simulink model "Speed_Controller_Test_gr3"  (Simulink 7.0)
settings: Solver=ode4  SolverMode=SingleTasking  StartTime=0.0  StopTime=252  FixedStep=0.01  RelTol=1e-3
InitFcn:
  | tempomat_para
StopFcn:
  | clear;
values from neighbouring files (symbols this model uses):
  A = 1.9    [tempomat_para.m]
  a_Fzg_max = 2    [tempomat_para.m]
  a_Fzg_min = -2    [tempomat_para.m]
  cw = 0.32    [tempomat_para.m]
  gang = [1 2 3 4]    [tempomat_para.m]
  gang_vec = [1 2 3 4]    [tempomat_para.m]
  i_anteil = 5    [tempomat_para.m]
  i_d = 3.42    [tempomat_para.m]
  i_g = [3.91 2.17 1.37 1.00]    [tempomat_para.m]
  lambda_gang = [1.3 1.25  1.17  1.05]    [tempomat_para.m]
  m_Fzg = 1400    [tempomat_para.m]
  M_mot_max = [130 149 163 170 168 166 162 158 150 139 123 80]    [tempomat_para.m]
  M_mot_min = [0 -40]    [tempomat_para.m]
  n_mot0 = 1000    [tempomat_para.m]
  n_mot_max = 1000:500:6500    [tempomat_para.m]
  n_mot_min = [1000 6500]    [tempomat_para.m]
  p_anteil = 100    [tempomat_para.m]
  r_dyn = 0.28    [tempomat_para.m]
  rho = 1.202    [tempomat_para.m]
  t_sch = 0.2    [tempomat_para.m]
  TI = [block '/TI']    [PSTI_callback.m]
  v_Fzg_ms0 = 0    [tempomat_para.m]
undefined symbols (not defined in the file or in its folder): Drossel_mat, getdatatypespecs
libraries: simulink x284, fzgbib x6
(part 1 of 19)
settings Model: Creator=Abel  LastModifiedBy=jza
settings DataIOCC: LimitDataPoints=off  SignalLoggingName=sigsOut
settings OptimizationCC: BooleanDataType=off
settings DebuggingCC: SaveWithParameterizedLinksMsg=none  SignalResolutionControl=TryResolveAllWithWarning  InheritedTsInSrcMsg=none  MultiTaskDSMMsg=warning  MultiTaskCondExecSysMsg=none  StrictBusMsg=None
settings RTWCC: IncludeERTFirstTime=on
settings GRTTargetCC: TargetFcnLib=ansi_tfl_tmw.mat

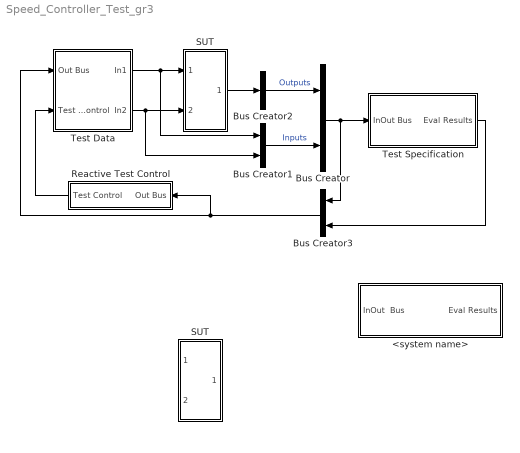
== system Speed_Controller_Test_gr3 ==
  <system name> : Subsystem  Description=Test evaluation system template. Create a new test evaluation system from this template.  mask{No=3, T=off}
      mask prompts: No "Number of Requirements"; T "Shut off the mask"
      mask StyleString: popup(1|2|3|4|5|6|7|8|9|10|11|12|13|14|15|16|17|18|19|20),checkbox
      mask CallbackString: system_name2(gcb);|shut_mask(gcb);
  Bus Creator : BusCreator  Inputs=2
  Bus Creator1 : BusCreator  Inputs=2
  Bus Creator2 : BusCreator  Inputs=1
  Bus Creator3 : BusCreator  Orientation=left  Inputs=2
  Reactive Test Control : Subsystem  Orientation=left
  SUT : Subsystem
  "SUT " : Subsystem
  Test Data : Subsystem
  Test Specification : Subsystem  Description=Test evaluation system template. Create a new test evaluation system from this template.
  wires:
  SUT/1(Out1) -> Bus Creator2/1
  Bus Creator/1 -> Test Specification/1(InOut Bus), Bus Creator3/1
  Bus Creator2/1 -> Bus Creator/1  "Outputs"
  Bus Creator1/1 -> Bus Creator/2  "Inputs"
  Bus Creator3/1 -> Test Data/1(Out Bus), Reactive Test Control/1(Out Bus)
  Test Specification/1(Eval Results) -> Bus Creator3/2
  Reactive Test Control/1(Test Control) -> Test Data/2(Test Control)
  Test Data/1(In1) -> SUT/1(In1), Bus Creator1/1
  Test Data/2(In2) -> SUT/2(In2), Bus Creator1/2

== system Speed_Controller_Test_gr3/<system name> ==
  InOut  Bus : Inport  OutDataType=sfix(16)  OutScaling=2^0
  <Requirement name> : Subsystem  Description=Requirement template. Create a new requirement from this template.  mask{No=1}
      mask prompts: No "Number of single Validation Functions"
      mask StyleString: popup(1|2|3|4|5|6|7|8|9|10|11|12|13|14|15|16|17|18|19|20)
      mask CallbackString: ReqName_callback(gcb);
  <Requirement name>2 : Subsystem  Description=Requirement template. Create a new requirement from this template.  mask{No=3}
      mask prompts: No "Number of single Validation Functions"
      mask StyleString: popup(1|2|3|4|5|6|7|8|9|10|11|12|13|14|15|16|17|18|19|20)
      mask CallbackString: ReqName_callback(gcb);
  <Requirement name>3 : Subsystem  Description=Requirement template. Create a new requirement from this template.  mask{No=2}
      mask prompts: No "Number of single Validation Functions"
      mask StyleString: popup(1|2|3|4|5|6|7|8|9|10|11|12|13|14|15|16|17|18|19|20)
      mask CallbackString: ReqName_callback(gcb);
  Arbitration : Subsystem
  Bus Creator : BusCreator  Inputs=3
  Bus Creator1 : BusCreator  Inputs=2
  Bus Creator4 : BusCreator  Inputs=6
  Bus Selector : BusSelector  OutputSignals=signal1.signal1.signal1,signal2.signal1.signal1,signal3.signal1.signal1,signal3.signal2.signal1,signal2.signal2.signal1,signal2.signal3.signal1
  Signal Conversion : SignalConversion  ConversionOutput=Bus copy
  Eval Results : Outport  OutDataType=sfix(16)  OutScaling=2^0
  wires:
  Bus Creator1/1 -> Eval Results/1
  Bus Creator4/1 -> Bus Creator1/2
  Signal Conversion/1 -> <Requirement name>/1(InOut Bus), <Requirement name>2/1(InOut Bus), <Requirement name>3/1(InOut Bus)
  InOut  Bus/1 -> Signal Conversion/1
  <Requirement name>/1(Test Info) -> Bus Creator/1
  Arbitration/1(OV) -> Bus Creator1/1
  <Requirement name>2/1(Test Info) -> Bus Creator/2
  <Requirement name>3/1(Test Info) -> Bus Creator/3
  Bus Creator/1 -> Bus Selector/1
  Bus Selector/1 -> Arbitration/1(v1), Bus Creator4/1  "<signal1>"
  Bus Selector/2 -> Arbitration/2(v2), Bus Creator4/2  "<signal1>"
  Bus Selector/3 -> Arbitration/3(v3), Bus Creator4/3  "<signal1>"
  Bus Selector/4 -> Arbitration/4(v4), Bus Creator4/4  "<signal1>"

== system Speed_Controller_Test_gr3/Reactive Test Control ==
  Out Bus : Inport  OutDataType=sfix(16)  OutScaling=2^0
  Bus Selector : BusSelector  OutputSignals=signal2.signal1.signal1.signal1.signal1.Local verdict
  Counter : Subsystem
  Memory : Memory
  OR : Logic  Operator=OR  Inputs=3  AllPortsSameDT=off  OutDataTypeMode=boolean
  Switch : Switch  Criteria=u2 > Threshold
  error : simulink/Logic and Bit Operations/Compare To Constant  SystemSampleTime=-1  relop===  const=-1  LogicOutDataTypeMode=uint8  ZeroCross=off
  fail : simulink/Logic and Bit Operations/Compare To Constant  SystemSampleTime=-1  relop===  const=0  LogicOutDataTypeMode=uint8  ZeroCross=off
  pass : simulink/Logic and Bit Operations/Compare To Constant  SystemSampleTime=-1  relop===  const=1  LogicOutDataTypeMode=uint8  ZeroCross=off
  test case 1 : Constant  OutDataType=sfix(16)  OutScaling=2^0
  test case 2 : Constant  Value=2  OutDataType=sfix(16)  OutScaling=2^0
  Test Control : Outport  OutDataType=sfix(16)  OutScaling=2^0
  wires:
  OR/1 -> Counter/1(In1), Counter/Trigger
  test case 1/1 -> Switch/3
  Out Bus/1 -> Bus Selector/1
  Switch/1 -> Test Control/1
  test case 2/1 -> Switch/1
  Counter/1(Out1) -> Switch/2
  Bus Selector/1 -> Memory/1  "<Local verdict>"
  pass/1 -> OR/1
  fail/1 -> OR/2
  error/1 -> OR/3
  Memory/1 -> pass/1, error/1, fail/1

== system Speed_Controller_Test_gr3/SUT ==
  In1 : Inport  OutDataType=sfix(16)  OutScaling=2^0
  In2 : Inport  Port=2  OutDataType=sfix(16)  OutScaling=2^0
  " Speed Controller " : Subsystem  AncestorBlock=fzgbib/GeschwindigkeitsRegelung
  Terminator1 : Terminator
  Terminator2 : Terminator
  Vehicle Model : Subsystem
      mask Type: Vehicle Model
      mask Display: image(imread('car.jpg','jpg'),[0.05,0.2,0.9,0.6])
  Out1 : Outport  OutDataType=sfix(16)  OutScaling=2^0
  wires:
  Vehicle Model/2(M_Br_b) -> Terminator1/1
  Vehicle Model/3(M_Mot_b) -> Terminator2/1
  " Speed Controller "/1(CarInputs) -> Vehicle Model/1(StellgroessenTempomat)
  Vehicle Model/1(FzgDaten) -> " Speed Controller "/1(CarOutputs)
  " Speed Controller "/2(v_act) -> Out1/1
  In2/1 -> " Speed Controller "/3(Selection)
  In1/1 -> " Speed Controller "/4(v_Des)

== system Speed_Controller_Test_gr3/SUT  ==
  In1 : Inport  OutDataType=sfix(16)  OutScaling=2^0
  In2 : Inport  Port=2  OutDataType=sfix(16)  OutScaling=2^0
  " Speed Controller " : Subsystem  AncestorBlock=fzgbib/GeschwindigkeitsRegelung
  Terminator1 : Terminator
  Terminator2 : Terminator
  Vehicle Model : Subsystem
      mask Type: Vehicle Model
      mask Display: image(imread('car.jpg','jpg'),[0.05,0.2,0.9,0.6])
  Out1 : Outport  OutDataType=sfix(16)  OutScaling=2^0
  wires:
  Vehicle Model/2(M_Br_b) -> Terminator1/1
  Vehicle Model/3(M_Mot_b) -> Terminator2/1
  " Speed Controller "/1(CarInputs) -> Vehicle Model/1(StellgroessenTempomat)
  Vehicle Model/1(FzgDaten) -> " Speed Controller "/1(CarOutputs)
  " Speed Controller "/2(v_act) -> Out1/1
  In2/1 -> " Speed Controller "/3(Selection)
  In1/1 -> " Speed Controller "/4(v_Des)

== system Speed_Controller_Test_gr3/Test Data ==
  Out Bus : Inport  OutDataType=sfix(16)  OutScaling=2^0
  Test Control : Inport  Port=2  OutDataType=sfix(16)  OutScaling=2^0
  Bus Creator : BusCreator  Inputs=6
  Bus Selector : BusSelector  OutputSignals=v_Des (signal 1),v_Des (signal 4)
  Bus Selector1 : BusSelector  OutputSignals=CCMode (signal 2),CCMode (signal 5)
  Bus Selector2 : BusSelector  OutputSignals=Selection (signal 3),Selection (signal 6)
  PrecAct CCMode : MultiPortSwitch  Inputs=3  zeroidx=on
  PrecAct Selection : MultiPortSwitch  Inputs=3  zeroidx=on
  PrecAct v_Des : MultiPortSwitch  Inputs=3  zeroidx=on
  R1 Speed Control step response : Subsystem
  R2 Speed Control velocity restoration time after simple  acceleration/deceleration : Subsystem
  zero signal : Constant  Value=0  OutDataType=sfix(16)  OutScaling=2^0
  In1 : Outport  OutDataType=sfix(16)  OutScaling=2^0
  In2 : Outport  Port=2  OutDataType=sfix(16)  OutScaling=2^0
  wires:
  Out Bus/1 -> R1 Speed Control step response/1(Out Bus)
  zero signal/1 -> PrecAct v_Des/2, PrecAct Selection/2, PrecAct CCMode/2
  PrecAct CCMode/1 -> In1/1
  PrecAct Selection/1 -> In2/1
  Bus Creator/1 -> Bus Selector/1, Bus Selector1/1, Bus Selector2/1
  Bus Selector/1 -> PrecAct v_Des/3  "<v_Des (signal 1)>"
  R1 Speed Control step response/1(v_Des) -> Bus Creator/1
  R1 Speed Control step response/2(CCMode) -> Bus Creator/2
  R1 Speed Control step response/3(Selection) -> Bus Creator/3
  R2 Speed Control velocity restoration time after simple  acceleration/deceleration/1(v_Des) -> Bus Creator/4
  R2 Speed Control velocity restoration time after simple  acceleration/deceleration/2(CCMode) -> Bus Creator/5
  R2 Speed Control velocity restoration time after simple  acceleration/deceleration/3(Selection) -> Bus Creator/6
  Bus Selector/2 -> PrecAct v_Des/4  "<v_Des (signal 4)>"
  Bus Selector1/1 -> PrecAct CCMode/3  "<CCMode (signal 2)>"
  Bus Selector1/2 -> PrecAct CCMode/4  "<CCMode (signal 5)>"
  Bus Selector2/1 -> PrecAct Selection/3  "<Selection (signal 3)>"
  Bus Selector2/2 -> PrecAct Selection/4  "<Selection (signal 6)>"
  Test Control/1 -> PrecAct v_Des/1, PrecAct CCMode/1, PrecAct Selection/1

== system Speed_Controller_Test_gr3/Test Specification ==
  InOut Bus : Inport  OutDataType=sfix(16)  OutScaling=2^0
  Arbitration : Subsystem
  Bus Creator1 : BusCreator  Inputs=2
  Bus Creator2 : BusCreator  Inputs=2
  Bus Selector1 : BusSelector  OutputSignals=signal1.signal1.signal1.Local verdict,signal1.signal1.signal2.Local verdict,signal2.signal1.signal1.Local verdict
  R1 Speed Control step response : Subsystem  Description=Requirement template. Create a new requirement from this template.
  R2 Speed Control velocity restoration time after simple  acceleration/deceleration : Subsystem  Description=Requirement template. Create a new requirement from this template.
  Signal Conversion : SignalConversion  ConversionOutput=Bus copy
  Eval Results : Outport  OutDataType=sfix(16)  OutScaling=2^0
  wires:
  Signal Conversion/1 -> R1 Speed Control step response/1(InOut Bus), R2 Speed Control velocity restoration time after simple  acceleration/deceleration/1(InOut Bus)
  R1 Speed Control step response/1(Test Info) -> Bus Creator2/1
  InOut Bus/1 -> Signal Conversion/1
  Bus Creator2/1 -> Bus Selector1/1, Bus Creator1/1
  R2 Speed Control velocity restoration time after simple  acceleration/deceleration/1(Test Info) -> Bus Creator2/2
  Bus Selector1/1 -> Arbitration/1(In1)  "<Local verdict>"
  Bus Selector1/2 -> Arbitration/2(In2)  "<Local verdict>"
  Bus Selector1/3 -> Arbitration/3(In3)  "<Local verdict>"
  Bus Creator1/1 -> Eval Results/1
  Arbitration/1(Out1) -> Bus Creator1/2  "Overall verdict"

== system Speed_Controller_Test_gr3/<system name>/<Requirement name> ==
  InOut Bus : Inport  OutDataType=sfix(16)  OutScaling=2^0
  <Assertions name> : Subsystem  Description=Assertions template. Create a new assertions block from this template.
  <Preconditions name> : Subsystem  Description=Preconditions template. Create new preconditions blocks using this template.
  Bus Creator : BusCreator  Inputs=1
  Test Info : Outport  OutDataType=sfix(16)  OutScaling=2^0
  wires:
  <Preconditions name>/1(Activate) -> <Assertions name>/1(Precond)
  Bus Creator/1 -> Test Info/1
  <Assertions name>/1(VF info) -> Bus Creator/1
  InOut Bus/1 -> <Preconditions name>/1(InOut Bus), <Assertions name>/2(InOut Bus)

== system Speed_Controller_Test_gr3/<system name>/<Requirement name>2 ==
  InOut Bus : Inport  OutDataType=sfix(16)  OutScaling=2^0
  <Assertions name> : Subsystem  Description=Assertions template. Create a new assertions block from this template.
  <Assertions name>2 : Subsystem  Description=Assertions template. Create a new assertions block from this template.
  <Assertions name>3 : Subsystem  Description=Assertions template. Create a new assertions block from this template.
  <Preconditions name> : Subsystem  Description=Preconditions template. Create new preconditions blocks using this template.
  <Preconditions name>2 : Subsystem  Description=Preconditions template. Create new preconditions blocks using this template.
  <Preconditions name>3 : Subsystem  Description=Preconditions template. Create new preconditions blocks using this template.
  Bus Creator : BusCreator  Inputs=3
  Test Info : Outport  OutDataType=sfix(16)  OutScaling=2^0
  wires:
  <Preconditions name>/1(Activate) -> <Assertions name>/1(Precond)
  Bus Creator/1 -> Test Info/1
  <Assertions name>/1(VF info) -> Bus Creator/1
  InOut Bus/1 -> <Preconditions name>/1(InOut Bus), <Assertions name>/2(InOut Bus), <Assertions name>2/2(InOut Bus), <Preconditions name>2/1(InOut Bus), <Assertions name>3/2(InOut Bus), <Preconditions name>3/1(InOut Bus)
  <Preconditions name>2/1(Activate) -> <Assertions name>2/1(Precond)
  <Assertions name>2/1(VF info) -> Bus Creator/2
  <Preconditions name>3/1(Activate) -> <Assertions name>3/1(Precond)
  <Assertions name>3/1(VF info) -> Bus Creator/3

== system Speed_Controller_Test_gr3/<system name>/<Requirement name>3 ==
  InOut Bus : Inport  OutDataType=sfix(16)  OutScaling=2^0
  <Assertions name> : Subsystem  Description=Assertions template. Create a new assertions block from this template.
  <Assertions name>2 : Subsystem  Description=Assertions template. Create a new assertions block from this template.
  <Preconditions name> : Subsystem  Description=Preconditions template. Create new preconditions blocks using this template.
  <Preconditions name>2 : Subsystem  Description=Preconditions template. Create new preconditions blocks using this template.
  Bus Creator : BusCreator  Inputs=2
  Test Info : Outport  OutDataType=sfix(16)  OutScaling=2^0
  wires:
  <Preconditions name>/1(Activate) -> <Assertions name>/1(Precond)
  Bus Creator/1 -> Test Info/1
  <Assertions name>/1(VF info) -> Bus Creator/1
  InOut Bus/1 -> <Preconditions name>/1(InOut Bus), <Assertions name>/2(InOut Bus), <Assertions name>2/2(InOut Bus), <Preconditions name>2/1(InOut Bus)
  <Preconditions name>2/1(Activate) -> <Assertions name>2/1(Precond)
  <Assertions name>2/1(VF info) -> Bus Creator/2

== system Speed_Controller_Test_gr3/<system name>/Arbitration ==
  v1 : Inport  OutDataType=sfix(16)  OutScaling=2^0
  v2 : Inport  Port=2  OutDataType=sfix(16)  OutScaling=2^0
  v3 : Inport  Port=3  OutDataType=sfix(16)  OutScaling=2^0
  v4 : Inport  Port=4  OutDataType=sfix(16)  OutScaling=2^0
  In1 : Inport  Port=5  OutDataType=sfix(16)  OutScaling=2^0
  In2 : Inport  Port=6  OutDataType=sfix(16)  OutScaling=2^0
  Collect Verdicts : MinMax  Inputs=3  OutDataType=sfix(16)  OutScaling=2^0
  Memory : Memory  Orientation=left  X0=2
  OV : Outport  OutDataType=sfix(16)  OutScaling=2^0
  wires:
  v1/1 -> Collect Verdicts/1
  Collect Verdicts/1 -> OV/1, Memory/1
  v2/1 -> Collect Verdicts/2
  v3/1 -> Collect Verdicts/3
  Memory/1 -> ?
  v4/1 -> ?

== system Speed_Controller_Test_gr3/Reactive Test Control/Counter ==
  In1 : Inport  OutDataType=sfix(16)  OutScaling=2^0
  Trigger : TriggerPort
  " 1" : DataTypeConversion  Orientation=down  OutDataType=sfix(16)  OutScaling=2^0
  Add : Sum  OutDataType=sfix(16)  OutScaling=2^-10
  Memory : Memory  Orientation=left  InheritSampleTime=on
  Number of triggers : Constant  Value=2  OutDataType=sfix(16)  OutScaling=2^0
  Relational Operator1 : RelationalOperator  Operator===  LogicOutDataTypeMode=boolean
  Scope1 : Scope  NumInputPorts=4
      settings: YMin=182.932~-5~-5~-5  YMax=202.188~5~5~5  SaveName=ScopeData14  MaxDataPoints=5000000
  Out1 : Outport  OutDataType=sfix(16)  OutScaling=2^0
  wires:
  In1/1 -> Add/1, Scope1/2
  Number of triggers/1 -> Relational Operator1/2
  Relational Operator1/1 -> Out1/1
  Add/1 -> " 1"/1, Relational Operator1/1, Scope1/3
  Memory/1 -> Add/2
  " 1"/1 -> Memory/1

== system Speed_Controller_Test_gr3/SUT/ Speed Controller  ==
  CarOutputs : Inport  OutDataType=sfix(16)  OutScaling=2^0
  CCMode : Inport  Port=2  OutDataType=sfix(16)  OutScaling=2^0
  Selection : Inport  Port=3  OutDataType=sfix(16)  OutScaling=2^0
  v_Des : Inport  Port=4  OutDataType=sfix(16)  OutScaling=2^0
  Bus Selector : BusSelector  OutputSignals=i_Total,n_Eng,a_Vhcl,v_act
  Compute SUC inputs : Subsystem  AncestorBlock=fzgbib/StellgroessenBerechnung BeschleunigungsBegrenzung
  Speed Controller : Subsystem  AncestorBlock=fzgbib/GeschwindigkeitsRegelung
  "km/h -> m/s2" : Gain  Gain=1/3.6  ParameterDataType=sfix(16)  ParameterScaling=2^0  OutDataType=sfix(16)  OutScaling=2^0  SaturateOnIntegerOverflow=on
  "m/s2 -> km/h" : Gain  Gain=3.6  ParameterDataType=sfix(16)  ParameterScaling=2^0  OutDataType=sfix(16)  OutScaling=2^0  SaturateOnIntegerOverflow=on
  CarInputs : Outport  OutDataType=sfix(16)  OutScaling=2^0
  v_act : Outport  Port=2  OutDataType=sfix(16)  OutScaling=2^0
  wires:
  Speed Controller/1(T) -> Compute SUC inputs/4(T)
  Bus Selector/1 -> Compute SUC inputs/1(i_Total)  "<i_Total>"
  Bus Selector/2 -> Compute SUC inputs/2(n_Eng)  "<n_Eng>"
  Bus Selector/3 -> Compute SUC inputs/3(a_Vhcl)  "<a_Vhcl>"
  Bus Selector/4 -> Speed Controller/1(v_Vhcl), "m/s2 -> km/h"/1  "<v_act>"
  Compute SUC inputs/1(SUC inputs) -> CarInputs/1
  v_Des/1 -> "km/h -> m/s2"/1
  "km/h -> m/s2"/1 -> Speed Controller/2(v_Des)
  Selection/1 -> Speed Controller/3(Selection)
  CCMode/1 -> Speed Controller/4(CCMode)
  CarOutputs/1 -> Bus Selector/1
  "m/s2 -> km/h"/1 -> v_act/1

== system Speed_Controller_Test_gr3/SUT/Vehicle Model ==
  note: i_Gesamt
      | n_mot
      | a_Fzg_mss
      | v_Fzg_ms
      | Gang_i
  StellgroessenTempomat : Inport  Orientation=left  OutDataType=sfix(16)  OutScaling=2^0
  Bremsmomenten beschaenkung : fzgbib/Bremsmomenten beschraenkung  Orientation=left  SystemSampleTime=-1
  Bus Creator : BusCreator  Orientation=left  Inputs=5
  Const : Constant  OutDataType=sfix(16)  OutScaling=2^0
  Fahrzeugmodell : Subsystem  Orientation=left  AncestorBlock=fzgbib/Fahrzeugmodell
  Gangberechnung : fzgbib/Gangberechnung  Orientation=left  SystemSampleTime=-1
  M_Mot M_Br : Demux  Orientation=left  Outputs=2
  Motormoment beschraenkung : fzgbib/Motormoment beschraenkung  Orientation=left  SystemSampleTime=-1
  SG-Koordinator : Subsystem  Orientation=left
  Terminator : Terminator
  FzgDaten : Outport  Orientation=left  OutDataType=sfix(16)  OutScaling=2^0
  M_Br_b : Outport  Orientation=left  Port=2  OutDataType=sfix(16)  OutScaling=2^0
  M_Mot_b : Outport  Orientation=left  Port=3  OutDataType=sfix(16)  OutScaling=2^0
  wires:
  M_Mot M_Br/1 -> Gangberechnung/1, Motormoment beschraenkung/1
  Fahrzeugmodell/5(a_Fzg_mss) -> Bus Creator/3  "a_Vhcl"
  Fahrzeugmodell/1(v_Fzg_ms) -> Bus Creator/4  "v_act"
  Motormoment beschraenkung/1 -> Fahrzeugmodell/2(M_Mot_b), M_Mot_b/1
  M_Mot M_Br/2 -> Bremsmomenten beschaenkung/1
  Fahrzeugmodell/4(Gang_i) -> Gangberechnung/3, Bus Creator/5  "Gang_i"
  Fahrzeugmodell/6("DK_Stellung ") -> Terminator/1
  Fahrzeugmodell/3(n_Mot) -> Gangberechnung/2, Motormoment beschraenkung/2, Bus Creator/2  "n_Eng"
  Fahrzeugmodell/2(i_gesamt) -> Bus Creator/1  "i_Total"
  Gangberechnung/1 -> Fahrzeugmodell/3(Gang_w)
  SG-Koordinator/1(Momente) -> M_Mot M_Br/1
  Bremsmomenten beschaenkung/1 -> Fahrzeugmodell/1(M_Br_b), M_Br_b/1
  StellgroessenTempomat/1 -> SG-Koordinator/1(Tempomat), SG-Koordinator/3(Fahrer)
  Const/1 -> SG-Koordinator/2(TempomatFlag)
  Bus Creator/1 -> FzgDaten/1

== system Speed_Controller_Test_gr3/SUT / Speed Controller  ==
  CarOutputs : Inport  OutDataType=sfix(16)  OutScaling=2^0
  CCMode : Inport  Port=2  OutDataType=sfix(16)  OutScaling=2^0
  Selection : Inport  Port=3  OutDataType=sfix(16)  OutScaling=2^0
  v_Des : Inport  Port=4  OutDataType=sfix(16)  OutScaling=2^0
  Bus Selector : BusSelector  OutputSignals=i_Total,n_Eng,a_Vhcl,v_act
  Compute SUC inputs : Subsystem  AncestorBlock=fzgbib/StellgroessenBerechnung BeschleunigungsBegrenzung
  Speed Controller : Subsystem  AncestorBlock=fzgbib/GeschwindigkeitsRegelung
  "km/h -> m/s2" : Gain  Gain=1/3.6  ParameterDataType=sfix(16)  ParameterScaling=2^0  OutDataType=sfix(16)  OutScaling=2^0  SaturateOnIntegerOverflow=on
  "m/s2 -> km/h" : Gain  Gain=3.6  ParameterDataType=sfix(16)  ParameterScaling=2^0  OutDataType=sfix(16)  OutScaling=2^0  SaturateOnIntegerOverflow=on
  CarInputs : Outport  OutDataType=sfix(16)  OutScaling=2^0
  v_act : Outport  Port=2  OutDataType=sfix(16)  OutScaling=2^0
  wires:
  Speed Controller/1(T) -> Compute SUC inputs/4(T)
  Bus Selector/1 -> Compute SUC inputs/1(i_Total)  "<i_Total>"
  Bus Selector/2 -> Compute SUC inputs/2(n_Eng)  "<n_Eng>"
  Bus Selector/3 -> Compute SUC inputs/3(a_Vhcl)  "<a_Vhcl>"
  Bus Selector/4 -> Speed Controller/1(v_Vhcl), "m/s2 -> km/h"/1  "<v_act>"
  Compute SUC inputs/1(SUC inputs) -> CarInputs/1
  v_Des/1 -> "km/h -> m/s2"/1
  "km/h -> m/s2"/1 -> Speed Controller/2(v_Des)
  Selection/1 -> Speed Controller/3(Selection)
  CCMode/1 -> Speed Controller/4(CCMode)
  CarOutputs/1 -> Bus Selector/1
  "m/s2 -> km/h"/1 -> v_act/1

== system Speed_Controller_Test_gr3/SUT /Vehicle Model ==
  note: i_Gesamt
      | n_mot
      | a_Fzg_mss
      | v_Fzg_ms
      | Gang_i
  StellgroessenTempomat : Inport  Orientation=left  OutDataType=sfix(16)  OutScaling=2^0
  Bremsmomenten beschaenkung : fzgbib/Bremsmomenten beschraenkung  Orientation=left  SystemSampleTime=-1
  Bus Creator : BusCreator  Orientation=left  Inputs=5
  Const : Constant  OutDataType=sfix(16)  OutScaling=2^0
  Fahrzeugmodell : Subsystem  Orientation=left  AncestorBlock=fzgbib/Fahrzeugmodell
  Gangberechnung : fzgbib/Gangberechnung  Orientation=left  SystemSampleTime=-1
  M_Mot M_Br : Demux  Orientation=left  Outputs=2
  Motormoment beschraenkung : fzgbib/Motormoment beschraenkung  Orientation=left  SystemSampleTime=-1
  SG-Koordinator : Subsystem  Orientation=left
  Terminator : Terminator
  FzgDaten : Outport  Orientation=left  OutDataType=sfix(16)  OutScaling=2^0
  M_Br_b : Outport  Orientation=left  Port=2  OutDataType=sfix(16)  OutScaling=2^0
  M_Mot_b : Outport  Orientation=left  Port=3  OutDataType=sfix(16)  OutScaling=2^0
  wires:
  M_Mot M_Br/1 -> Gangberechnung/1, Motormoment beschraenkung/1
  Fahrzeugmodell/5(a_Fzg_mss) -> Bus Creator/3  "a_Vhcl"
  Fahrzeugmodell/1(v_Fzg_ms) -> Bus Creator/4  "v_act"
  Motormoment beschraenkung/1 -> Fahrzeugmodell/2(M_Mot_b), M_Mot_b/1
  M_Mot M_Br/2 -> Bremsmomenten beschaenkung/1
  Fahrzeugmodell/4(Gang_i) -> Gangberechnung/3, Bus Creator/5  "Gang_i"
  Fahrzeugmodell/6("DK_Stellung ") -> Terminator/1
  Fahrzeugmodell/3(n_Mot) -> Gangberechnung/2, Motormoment beschraenkung/2, Bus Creator/2  "n_Eng"
  Fahrzeugmodell/2(i_gesamt) -> Bus Creator/1  "i_Total"
  Gangberechnung/1 -> Fahrzeugmodell/3(Gang_w)
  SG-Koordinator/1(Momente) -> M_Mot M_Br/1
  Bremsmomenten beschaenkung/1 -> Fahrzeugmodell/1(M_Br_b), M_Br_b/1
  StellgroessenTempomat/1 -> SG-Koordinator/1(Tempomat), SG-Koordinator/3(Fahrer)
  Const/1 -> SG-Koordinator/2(TempomatFlag)
  Bus Creator/1 -> FzgDaten/1

== system Speed_Controller_Test_gr3/Test Data/R1 Speed Control step response ==
  Out Bus : Inport  OutDataType=sfix(16)  OutScaling=2^0
  Complete step & CC active + no target & Speed Control active : Subsystem  Description=Preconditions template. Create new preconditions blocks using this template.
  v_Des : Outport  OutDataType=sfix(16)  OutScaling=2^0
  CCMode : Outport  Port=2  OutDataType=sfix(16)  OutScaling=2^0
  Selection : Outport  Port=3  OutDataType=sfix(16)  OutScaling=2^0
  wires:
  Complete step & CC active + no target & Speed Control active/1(v_Des) -> v_Des/1  "v_Des"
  Complete step & CC active + no target & Speed Control active/2(CCMode) -> CCMode/1  "CCMode"
  Complete step & CC active + no target & Speed Control active/3(Selection) -> Selection/1  "Selection"
  Out Bus/1 -> Complete step & CC active + no target & Speed Control active/1(Out Bus)

== system Speed_Controller_Test_gr3/Test Data/R2 Speed Control velocity restoration time after simple  acceleration/deceleration ==
  " CC active + no target & Speed Control active & V_Des increases/decreases  7 times by 1 unit" : Subsystem  Description=Preconditions template. Create new preconditions blocks using this template.
  v_Des : Outport  OutDataType=sfix(16)  OutScaling=2^0
  CCMode : Outport  Port=2  OutDataType=sfix(16)  OutScaling=2^0
  Selection : Outport  Port=3  OutDataType=sfix(16)  OutScaling=2^0
  wires:
  " CC active + no target & Speed Control active & V_Des increases/decreases  7 times by 1 unit"/2(CCMode) -> CCMode/1  "CCMode"
  " CC active + no target & Speed Control active & V_Des increases/decreases  7 times by 1 unit"/3(Selection) -> Selection/1  "Selection"
  " CC active + no target & Speed Control active & V_Des increases/decreases  7 times by 1 unit"/1(v_Des) -> v_Des/1  "v_Des"

== system Speed_Controller_Test_gr3/Test Specification/Arbitration ==
  In1 : Inport  OutDataType=sfix(16)  OutScaling=2^0
  In2 : Inport  Port=2  OutDataType=sfix(16)  OutScaling=2^0
  In3 : Inport  Port=3  OutDataType=sfix(16)  OutScaling=2^0
  Collect Verdicts : MinMax  Inputs=4  OutDataType=sfix(16)  OutScaling=2^0
  Memory : Memory  Orientation=left  X0=2
  Out1 : Outport  OutDataType=sfix(16)  OutScaling=2^0
  wires:
  Memory/1 -> Collect Verdicts/4
  Collect Verdicts/1 -> Out1/1, Memory/1
  In1/1 -> Collect Verdicts/1
  In2/1 -> Collect Verdicts/2
  In3/1 -> Collect Verdicts/3

== system Speed_Controller_Test_gr3/Test Specification/R1 Speed Control step response ==
  InOut Bus : Inport  OutDataType=sfix(16)  OutScaling=2^0
  Bus Creator : BusCreator  Inputs=2
  Complete step & CC active + no target & Speed Control active : Subsystem  Description=Preconditions template. Create new preconditions blocks using this template.
  Maximum overshoot < 5 &  Steady state error < 5 : Subsystem  Description=Assertions template. Create a new assertions block from this template.
  Test Info : Outport  OutDataType=sfix(16)  OutScaling=2^0
  wires:
  InOut Bus/1 -> Complete step & CC active + no target & Speed Control active/1(InOut Bus), Maximum overshoot < 5 &  Steady state error < 5/2(InOut Bus)
  Maximum overshoot < 5 &  Steady state error < 5/1(VF info) -> Bus Creator/1
  Bus Creator/1 -> Test Info/1
  Complete step & CC active + no target & Speed Control active/1(Activate) -> Maximum overshoot < 5 &  Steady state error < 5/1(Precond), Bus Creator/2

== system Speed_Controller_Test_gr3/Test Specification/R2 Speed Control velocity restoration time after simple  acceleration/deceleration ==
  InOut Bus : Inport  OutDataType=sfix(16)  OutScaling=2^0
  Bus Creator : BusCreator  Inputs=2
  CC active + no target & Speed Control active & step of V_Des = |1|  with time periods >= 7s : Subsystem  Description=Preconditions template. Create new preconditions blocks using this template.
  after (6 seconds)  |V_Des-V_Vhcl <= 1.4| : Subsystem  Description=Assertions template. Create a new assertions block from this template.
  Test Info : Outport  OutDataType=sfix(16)  OutScaling=2^0
  wires:
  InOut Bus/1 -> CC active + no target & Speed Control active & step of V_Des = |1|  with time periods >= 7s/1(InOut Bus), after (6 seconds)  |V_Des-V_Vhcl <= 1.4|/2(InOut Bus)
  after (6 seconds)  |V_Des-V_Vhcl <= 1.4|/1(VF info) -> Bus Creator/1
  Bus Creator/1 -> Test Info/1
  CC active + no target & Speed Control active & step of V_Des = |1|  with time periods >= 7s/1(Activate) -> after (6 seconds)  |V_Des-V_Vhcl <= 1.4|/1(Precond), Bus Creator/2

== system Speed_Controller_Test_gr3/<system name>/<Requirement name>/<Assertions name> ==
  Precond : Inport  OutDataType=sfix(16)  OutScaling=2^0
  InOut Bus : Inport  Port=2  OutDataType=sfix(16)  OutScaling=2^0
  <Reference name> : Constant  OutDataType=sfix(16)  OutScaling=2^0
  Bus Creator : BusCreator  Inputs=1
  Bus Selector : BusSelector  OutputSignals=signal1
  Feature extraction : Subsystem  TreatAsAtomicUnit=on  mask{Param=0}
      mask prompts: Param "Mask Parameter 1:"
  PAS : Subsystem  mask{AFT=TID, AFD=600}
      mask prompts: AFT "Assertion feature type:"; AFD "Assertion feature delay (in time steps)"
      mask init:
      | PAS_init(gcb);
      mask StyleString: popup(TI|TDD|TID),edit
      mask CallbackString: PAS_callback(gcb);|
  Signal comparison : Subsystem  TreatAsAtomicUnit=on  mask{Param=0}
      mask prompts: Param "Mask Parameter 1:"
  VF info : Outport  OutDataType=sfix(16)  OutScaling=2^0
  wires:
  Bus Creator/1 -> VF info/1
  InOut Bus/1 -> Bus Selector/1
  Precond/1 -> PAS/1(Precond)
  PAS/1(VF Info) -> Bus Creator/1
  <Reference name>/1 -> Signal comparison/2(Ref)
  Feature extraction/3(A) -> Signal comparison/1(Sig)
  Feature extraction/2(T) -> PAS/3(T)
  Feature extraction/1(R) -> PAS/2(R)
  Bus Selector/1 -> Feature extraction/1(Sig)  "<signal1>"
  Signal comparison/1(V) -> PAS/4(V)

== system Speed_Controller_Test_gr3/<system name>/<Requirement name>/<Preconditions name> ==
  InOut Bus : Inport  OutDataType=sfix(16)  OutScaling=2^0
  <Reference name> : Constant  OutDataType=sfix(16)  OutScaling=2^0
  Bus Selector : BusSelector  OutputSignals=signal1
  Feature extraction : Subsystem  TreatAsAtomicUnit=on  mask{Param=0}
      mask prompts: Param "Mask Parameter 1:"
  PS : Subsystem  mask(Feature layer: preconditions synchronization){NoTI=0, NoTDD=0, NoTID=1, TIdel=[0], TDDdel=[0]}
      mask prompts: NoTI "Time-independent features identifiable with or without a delay (TI)"; NoTDD "Triggered features identifiable with determinate delay or without a delay (TDD)"; NoTID "Triggered features identifiable with indeterminate delay (TID)"; TIdel "Time-independent features delays (in time steps). E.g. [0 1 0] for 3 features"; TDDdel "Triggered features delays (in time steps). E.g. [0 0] for 2 features"
      mask help: Use this block for synchronizing the precondition features. For changing the block inputs, use the parameters below. The output must be used for assertions activation.
      mask init:
      | PS_init(gcb);
      mask StyleString: popup(0|1|2|3|4|5|6|7|8|9),popup(0|1|2|3|4|5|6|7|8|9),popup(0|1|2|3|4|5|6|7|8|9),edit,edit
      mask CallbackString:
      | PSTI_callback(gcb);|PSTDD_callback(gcb);|PSTID_callback(gcb);|NoTI = str2double(get_param(gcb,'NoTI'));
      | TIdel = str2num(get_param(gcb,'TIdel'));
      | if NoTI ~= length(TIdel) && NoTI ~= 0
      |     error(['The number of delays entered (' num2str(length(TIdel)) ') does not correspond to the above specified number of time-independent features (' num2str(NoTI) ').']);
      | end|NoTDD = str2double(get_param(gcb,'NoTDD'));
      | TDDdel = str2num(get_param(gcb,'TDDdel'));
      | if NoTDD ~= length(TDDdel) && NoTDD ~= 0
      |     error(['The number of delays entered (' num2str(length(TDDdel)) ') does not correspond to the above specified number of triggered features with constant delay (' num2str(NoTDD) ').']);
      | end
  Signal comparison : Subsystem  TreatAsAtomicUnit=on  mask{Param=0}
      mask prompts: Param "Mask Parameter 1:"
  Activate : Outport  OutDataType=sfix(16)  OutScaling=2^0
  wires:
  InOut Bus/1 -> Bus Selector/1
  PS/1(Precond) -> Activate/1
  Signal comparison/1(A) -> PS/3(A TID1)
  <Reference name>/1 -> Signal comparison/2(Ref)
  Feature extraction/3(A) -> Signal comparison/1(Sig)
  Feature extraction/2(T) -> PS/2(T TID1)
  Feature extraction/1(R) -> PS/1(R TID1)
  Bus Selector/1 -> Feature extraction/1(Sig)  "<signal1>"

== system Speed_Controller_Test_gr3/<system name>/<Requirement name>2/<Assertions name> ==
  Precond : Inport  OutDataType=sfix(16)  OutScaling=2^0
  InOut Bus : Inport  Port=2  OutDataType=sfix(16)  OutScaling=2^0
  <Reference name> : Constant  OutDataType=sfix(16)  OutScaling=2^0
  Bus Creator : BusCreator  Inputs=1
  Bus Selector : BusSelector  OutputSignals=signal1
  Feature extraction : Subsystem  TreatAsAtomicUnit=on  mask{Param=0}
      mask prompts: Param "Mask Parameter 1:"
  PAS : Subsystem  mask{AFT=TID, AFD=600}
      mask prompts: AFT "Assertion feature type:"; AFD "Assertion feature delay (in time steps)"
      mask init:
      | PAS_init(gcb);
      mask StyleString: popup(TI|TDD|TID),edit
      mask CallbackString: PAS_callback(gcb);|
  Signal comparison : Subsystem  TreatAsAtomicUnit=on  mask{Param=0}
      mask prompts: Param "Mask Parameter 1:"
  VF info : Outport  OutDataType=sfix(16)  OutScaling=2^0
  wires:
  Bus Creator/1 -> VF info/1
  InOut Bus/1 -> Bus Selector/1
  Precond/1 -> PAS/1(Precond)
  PAS/1(VF Info) -> Bus Creator/1
  <Reference name>/1 -> Signal comparison/2(Ref)
  Feature extraction/3(A) -> Signal comparison/1(Sig)
  Feature extraction/2(T) -> PAS/3(T)
  Feature extraction/1(R) -> PAS/2(R)
  Bus Selector/1 -> Feature extraction/1(Sig)  "<signal1>"
  Signal comparison/1(V) -> PAS/4(V)

== system Speed_Controller_Test_gr3/<system name>/<Requirement name>2/<Assertions name>2 ==
  Precond : Inport  OutDataType=sfix(16)  OutScaling=2^0
  InOut Bus : Inport  Port=2  OutDataType=sfix(16)  OutScaling=2^0
  <Reference name> : Constant  OutDataType=sfix(16)  OutScaling=2^0
  Bus Creator : BusCreator  Inputs=1
  Bus Selector : BusSelector  OutputSignals=signal1
  Feature extraction : Subsystem  TreatAsAtomicUnit=on  mask{Param=0}
      mask prompts: Param "Mask Parameter 1:"
  PAS : Subsystem  mask{AFT=TID, AFD=600}
      mask prompts: AFT "Assertion feature type:"; AFD "Assertion feature delay (in time steps)"
      mask init:
      | PAS_init(gcb);
      mask StyleString: popup(TI|TDD|TID),edit
      mask CallbackString: PAS_callback(gcb);|
  Signal comparison : Subsystem  TreatAsAtomicUnit=on  mask{Param=0}
      mask prompts: Param "Mask Parameter 1:"
  VF info : Outport  OutDataType=sfix(16)  OutScaling=2^0
  wires:
  Bus Creator/1 -> VF info/1
  InOut Bus/1 -> Bus Selector/1
  Precond/1 -> PAS/1(Precond)
  PAS/1(VF Info) -> Bus Creator/1
  <Reference name>/1 -> Signal comparison/2(Ref)
  Feature extraction/3(A) -> Signal comparison/1(Sig)
  Feature extraction/2(T) -> PAS/3(T)
  Feature extraction/1(R) -> PAS/2(R)
  Bus Selector/1 -> Feature extraction/1(Sig)  "<signal1>"
  Signal comparison/1(V) -> PAS/4(V)

== system Speed_Controller_Test_gr3/<system name>/<Requirement name>2/<Assertions name>3 ==
  Precond : Inport  OutDataType=sfix(16)  OutScaling=2^0
  InOut Bus : Inport  Port=2  OutDataType=sfix(16)  OutScaling=2^0
  <Reference name> : Constant  OutDataType=sfix(16)  OutScaling=2^0
  Bus Creator : BusCreator  Inputs=1
  Bus Selector : BusSelector  OutputSignals=signal1
  Feature extraction : Subsystem  TreatAsAtomicUnit=on  mask{Param=0}
      mask prompts: Param "Mask Parameter 1:"
  PAS : Subsystem  mask{AFT=TID, AFD=600}
      mask prompts: AFT "Assertion feature type:"; AFD "Assertion feature delay (in time steps)"
      mask init:
      | PAS_init(gcb);
      mask StyleString: popup(TI|TDD|TID),edit
      mask CallbackString: PAS_callback(gcb);|
  Signal comparison : Subsystem  TreatAsAtomicUnit=on  mask{Param=0}
      mask prompts: Param "Mask Parameter 1:"
  VF info : Outport  OutDataType=sfix(16)  OutScaling=2^0
  wires:
  Bus Creator/1 -> VF info/1
  InOut Bus/1 -> Bus Selector/1
  Precond/1 -> PAS/1(Precond)
  PAS/1(VF Info) -> Bus Creator/1
  <Reference name>/1 -> Signal comparison/2(Ref)
  Feature extraction/3(A) -> Signal comparison/1(Sig)
  Feature extraction/2(T) -> PAS/3(T)
  Feature extraction/1(R) -> PAS/2(R)
  Bus Selector/1 -> Feature extraction/1(Sig)  "<signal1>"
  Signal comparison/1(V) -> PAS/4(V)

== system Speed_Controller_Test_gr3/<system name>/<Requirement name>2/<Preconditions name> ==
  InOut Bus : Inport  OutDataType=sfix(16)  OutScaling=2^0
  <Reference name> : Constant  OutDataType=sfix(16)  OutScaling=2^0
  Bus Selector : BusSelector  OutputSignals=signal1
  Feature extraction : Subsystem  TreatAsAtomicUnit=on  mask{Param=0}
      mask prompts: Param "Mask Parameter 1:"
  PS : Subsystem  mask(Feature layer: preconditions synchronization){NoTI=0, NoTDD=0, NoTID=1, TIdel=[], TDDdel=[]}
      mask prompts: NoTI "Time-independent features identifiable with or without a delay (TI)"; NoTDD "Triggered features identifiable with determinate delay or without a delay (TDD)"; NoTID "Triggered features identifiable with indeterminate delay (TID)"; TIdel "Time-independent features delays (in time steps). E.g. [0 1 0] for 3 features"; TDDdel "Triggered features delays (in time steps). E.g. [0 0] for 2 features"
      mask help: Use this block for synchronizing the precondition features. For changing the block inputs, use the parameters below. The output must be used for assertions activation.
      mask init:
      | PS_init(gcb);
      mask StyleString: popup(0|1|2|3|4|5|6|7|8|9),popup(0|1|2|3|4|5|6|7|8|9),popup(0|1|2|3|4|5|6|7|8|9),edit,edit
      mask CallbackString:
      | PSTI_callback(gcb);|PSTDD_callback(gcb);|PSTID_callback(gcb);|NoTI = str2double(get_param(gcb,'NoTI'));
      | TIdel = str2num(get_param(gcb,'TIdel'));
      | if NoTI ~= length(TIdel) && NoTI ~= 0
      |     error(['The number of delays entered (' num2str(length(TIdel)) ') does not correspond to the above specified number of time-independent features (' num2str(NoTI) ').']);
      | end|NoTDD = str2double(get_param(gcb,'NoTDD'));
      | TDDdel = str2num(get_param(gcb,'TDDdel'));
      | if NoTDD ~= length(TDDdel) && NoTDD ~= 0
      |     error(['The number of delays entered (' num2str(length(TDDdel)) ') does not correspond to the above specified number of triggered features with constant delay (' num2str(NoTDD) ').']);
      | end
  Signal comparison : Subsystem  TreatAsAtomicUnit=on  mask{Param=0}
      mask prompts: Param "Mask Parameter 1:"
  Activate : Outport  OutDataType=sfix(16)  OutScaling=2^0
  wires:
  InOut Bus/1 -> Bus Selector/1
  PS/1(Precond) -> Activate/1
  Signal comparison/1(A) -> PS/3(A TID1)
  <Reference name>/1 -> Signal comparison/2(Ref)
  Feature extraction/3(A) -> Signal comparison/1(Sig)
  Feature extraction/2(T) -> PS/2(T TID1)
  Feature extraction/1(R) -> PS/1(R TID1)
  Bus Selector/1 -> Feature extraction/1(Sig)  "<signal1>"

== system Speed_Controller_Test_gr3/<system name>/<Requirement name>2/<Preconditions name>2 ==
  InOut Bus : Inport  OutDataType=sfix(16)  OutScaling=2^0
  <Reference name> : Constant  OutDataType=sfix(16)  OutScaling=2^0
  Bus Selector : BusSelector  OutputSignals=signal1
  Feature extraction : Subsystem  TreatAsAtomicUnit=on  mask{Param=0}
      mask prompts: Param "Mask Parameter 1:"
  PS : Subsystem  mask(Feature layer: preconditions synchronization){NoTI=0, NoTDD=0, NoTID=1, TIdel=[0], TDDdel=[0]}
      mask prompts: NoTI "Time-independent features identifiable with or without a delay (TI)"; NoTDD "Triggered features identifiable with determinate delay or without a delay (TDD)"; NoTID "Triggered features identifiable with indeterminate delay (TID)"; TIdel "Time-independent features delays (in time steps). E.g. [0 1 0] for 3 features"; TDDdel "Triggered features delays (in time steps). E.g. [0 0] for 2 features"
      mask help: Use this block for synchronizing the precondition features. For changing the block inputs, use the parameters below. The output must be used for assertions activation.
      mask init:
      | PS_init(gcb);
      mask StyleString: popup(0|1|2|3|4|5|6|7|8|9),popup(0|1|2|3|4|5|6|7|8|9),popup(0|1|2|3|4|5|6|7|8|9),edit,edit
      mask CallbackString:
      | PSTI_callback(gcb);|PSTDD_callback(gcb);|PSTID_callback(gcb);|NoTI = str2double(get_param(gcb,'NoTI'));
      | TIdel = str2num(get_param(gcb,'TIdel'));
      | if NoTI ~= length(TIdel) && NoTI ~= 0
      |     error(['The number of delays entered (' num2str(length(TIdel)) ') does not correspond to the above specified number of time-independent features (' num2str(NoTI) ').']);
      | end|NoTDD = str2double(get_param(gcb,'NoTDD'));
      | TDDdel = str2num(get_param(gcb,'TDDdel'));
      | if NoTDD ~= length(TDDdel) && NoTDD ~= 0
      |     error(['The number of delays entered (' num2str(length(TDDdel)) ') does not correspond to the above specified number of triggered features with constant delay (' num2str(NoTDD) ').']);
      | end
  Signal comparison : Subsystem  TreatAsAtomicUnit=on  mask{Param=0}
      mask prompts: Param "Mask Parameter 1:"
  Activate : Outport  OutDataType=sfix(16)  OutScaling=2^0
  wires:
  InOut Bus/1 -> Bus Selector/1
  PS/1(Precond) -> Activate/1
  Signal comparison/1(A) -> PS/3(A TID1)
  <Reference name>/1 -> Signal comparison/2(Ref)
  Feature extraction/3(A) -> Signal comparison/1(Sig)
  Feature extraction/2(T) -> PS/2(T TID1)
  Feature extraction/1(R) -> PS/1(R TID1)
  Bus Selector/1 -> Feature extraction/1(Sig)  "<signal1>"

== system Speed_Controller_Test_gr3/<system name>/<Requirement name>2/<Preconditions name>3 ==
  InOut Bus : Inport  OutDataType=sfix(16)  OutScaling=2^0
  <Reference name> : Constant  OutDataType=sfix(16)  OutScaling=2^0
  Bus Selector : BusSelector  OutputSignals=signal1
  Feature extraction : Subsystem  TreatAsAtomicUnit=on  mask{Param=0}
      mask prompts: Param "Mask Parameter 1:"
  PS : Subsystem  mask(Feature layer: preconditions synchronization){NoTI=0, NoTDD=0, NoTID=1, TIdel=[0], TDDdel=[0]}
      mask prompts: NoTI "Time-independent features identifiable with or without a delay (TI)"; NoTDD "Triggered features identifiable with determinate delay or without a delay (TDD)"; NoTID "Triggered features identifiable with indeterminate delay (TID)"; TIdel "Time-independent features delays (in time steps). E.g. [0 1 0] for 3 features"; TDDdel "Triggered features delays (in time steps). E.g. [0 0] for 2 features"
      mask help: Use this block for synchronizing the precondition features. For changing the block inputs, use the parameters below. The output must be used for assertions activation.
      mask init:
      | PS_init(gcb);
      mask StyleString: popup(0|1|2|3|4|5|6|7|8|9),popup(0|1|2|3|4|5|6|7|8|9),popup(0|1|2|3|4|5|6|7|8|9),edit,edit
      mask CallbackString:
      | PSTI_callback(gcb);|PSTDD_callback(gcb);|PSTID_callback(gcb);|NoTI = str2double(get_param(gcb,'NoTI'));
      | TIdel = str2num(get_param(gcb,'TIdel'));
      | if NoTI ~= length(TIdel) && NoTI ~= 0
      |     error(['The number of delays entered (' num2str(length(TIdel)) ') does not correspond to the above specified number of time-independent features (' num2str(NoTI) ').']);
      | end|NoTDD = str2double(get_param(gcb,'NoTDD'));
      | TDDdel = str2num(get_param(gcb,'TDDdel'));
      | if NoTDD ~= length(TDDdel) && NoTDD ~= 0
      |     error(['The number of delays entered (' num2str(length(TDDdel)) ') does not correspond to the above specified number of triggered features with constant delay (' num2str(NoTDD) ').']);
      | end
  Signal comparison : Subsystem  TreatAsAtomicUnit=on  mask{Param=0}
      mask prompts: Param "Mask Parameter 1:"
  Activate : Outport  OutDataType=sfix(16)  OutScaling=2^0
  wires:
  InOut Bus/1 -> Bus Selector/1
  PS/1(Precond) -> Activate/1
  Signal comparison/1(A) -> PS/3(A TID1)
  <Reference name>/1 -> Signal comparison/2(Ref)
  Feature extraction/3(A) -> Signal comparison/1(Sig)
  Feature extraction/2(T) -> PS/2(T TID1)
  Feature extraction/1(R) -> PS/1(R TID1)
  Bus Selector/1 -> Feature extraction/1(Sig)  "<signal1>"

== system Speed_Controller_Test_gr3/<system name>/<Requirement name>3/<Assertions name> ==
  Precond : Inport  OutDataType=sfix(16)  OutScaling=2^0
  InOut Bus : Inport  Port=2  OutDataType=sfix(16)  OutScaling=2^0
  <Reference name> : Constant  OutDataType=sfix(16)  OutScaling=2^0
  Bus Creator : BusCreator  Inputs=1
  Bus Selector : BusSelector  OutputSignals=signal1
  Feature extraction : Subsystem  TreatAsAtomicUnit=on  mask{Param=0}
      mask prompts: Param "Mask Parameter 1:"
  PAS : Subsystem  mask{AFT=TID, AFD=600}
      mask prompts: AFT "Assertion feature type:"; AFD "Assertion feature delay (in time steps)"
      mask init:
      | PAS_init(gcb);
      mask StyleString: popup(TI|TDD|TID),edit
      mask CallbackString: PAS_callback(gcb);|
  Signal comparison : Subsystem  TreatAsAtomicUnit=on  mask{Param=0}
      mask prompts: Param "Mask Parameter 1:"
  VF info : Outport  OutDataType=sfix(16)  OutScaling=2^0
  wires:
  Bus Creator/1 -> VF info/1
  InOut Bus/1 -> Bus Selector/1
  Precond/1 -> PAS/1(Precond)
  PAS/1(VF Info) -> Bus Creator/1
  <Reference name>/1 -> Signal comparison/2(Ref)
  Feature extraction/3(A) -> Signal comparison/1(Sig)
  Feature extraction/2(T) -> PAS/3(T)
  Feature extraction/1(R) -> PAS/2(R)
  Bus Selector/1 -> Feature extraction/1(Sig)  "<signal1>"
  Signal comparison/1(V) -> PAS/4(V)

== system Speed_Controller_Test_gr3/<system name>/<Requirement name>3/<Assertions name>2 ==
  Precond : Inport  OutDataType=sfix(16)  OutScaling=2^0
  InOut Bus : Inport  Port=2  OutDataType=sfix(16)  OutScaling=2^0
  <Reference name> : Constant  OutDataType=sfix(16)  OutScaling=2^0
  Bus Creator : BusCreator  Inputs=1
  Bus Selector : BusSelector  OutputSignals=signal1
  Feature extraction : Subsystem  TreatAsAtomicUnit=on  mask{Param=0}
      mask prompts: Param "Mask Parameter 1:"
  PAS : Subsystem  mask{AFT=TID, AFD=600}
      mask prompts: AFT "Assertion feature type:"; AFD "Assertion feature delay (in time steps)"
      mask init:
      | PAS_init(gcb);
      mask StyleString: popup(TI|TDD|TID),edit
      mask CallbackString: PAS_callback(gcb);|
  Signal comparison : Subsystem  TreatAsAtomicUnit=on  mask{Param=0}
      mask prompts: Param "Mask Parameter 1:"
  VF info : Outport  OutDataType=sfix(16)  OutScaling=2^0
  wires:
  Bus Creator/1 -> VF info/1
  InOut Bus/1 -> Bus Selector/1
  Precond/1 -> PAS/1(Precond)
  PAS/1(VF Info) -> Bus Creator/1
  <Reference name>/1 -> Signal comparison/2(Ref)
  Feature extraction/3(A) -> Signal comparison/1(Sig)
  Feature extraction/2(T) -> PAS/3(T)
  Feature extraction/1(R) -> PAS/2(R)
  Bus Selector/1 -> Feature extraction/1(Sig)  "<signal1>"
  Signal comparison/1(V) -> PAS/4(V)

== system Speed_Controller_Test_gr3/<system name>/<Requirement name>3/<Preconditions name> ==
  InOut Bus : Inport  OutDataType=sfix(16)  OutScaling=2^0
  <Reference name> : Constant  OutDataType=sfix(16)  OutScaling=2^0
  Bus Selector : BusSelector  OutputSignals=signal1
  Feature extraction : Subsystem  TreatAsAtomicUnit=on  mask{Param=0}
      mask prompts: Param "Mask Parameter 1:"
  PS : Subsystem  mask(Feature layer: preconditions synchronization){NoTI=0, NoTDD=0, NoTID=1, TIdel=[0], TDDdel=[0]}
      mask prompts: NoTI "Time-independent features identifiable with or without a delay (TI)"; NoTDD "Triggered features identifiable with determinate delay or without a delay (TDD)"; NoTID "Triggered features identifiable with indeterminate delay (TID)"; TIdel "Time-independent features delays (in time steps). E.g. [0 1 0] for 3 features"; TDDdel "Triggered features delays (in time steps). E.g. [0 0] for 2 features"
      mask help: Use this block for synchronizing the precondition features. For changing the block inputs, use the parameters below. The output must be used for assertions activation.
      mask init:
      | PS_init(gcb);
      mask StyleString: popup(0|1|2|3|4|5|6|7|8|9),popup(0|1|2|3|4|5|6|7|8|9),popup(0|1|2|3|4|5|6|7|8|9),edit,edit
      mask CallbackString:
      | PSTI_callback(gcb);|PSTDD_callback(gcb);|PSTID_callback(gcb);|NoTI = str2double(get_param(gcb,'NoTI'));
      | TIdel = str2num(get_param(gcb,'TIdel'));
      | if NoTI ~= length(TIdel) && NoTI ~= 0
      |     error(['The number of delays entered (' num2str(length(TIdel)) ') does not correspond to the above specified number of time-independent features (' num2str(NoTI) ').']);
      | end|NoTDD = str2double(get_param(gcb,'NoTDD'));
      | TDDdel = str2num(get_param(gcb,'TDDdel'));
      | if NoTDD ~= length(TDDdel) && NoTDD ~= 0
      |     error(['The number of delays entered (' num2str(length(TDDdel)) ') does not correspond to the above specified number of triggered features with constant delay (' num2str(NoTDD) ').']);
      | end
  Signal comparison : Subsystem  TreatAsAtomicUnit=on  mask{Param=0}
      mask prompts: Param "Mask Parameter 1:"
  Activate : Outport  OutDataType=sfix(16)  OutScaling=2^0
  wires:
  InOut Bus/1 -> Bus Selector/1
  PS/1(Precond) -> Activate/1
  Signal comparison/1(A) -> PS/3(A TID1)
  <Reference name>/1 -> Signal comparison/2(Ref)
  Feature extraction/3(A) -> Signal comparison/1(Sig)
  Feature extraction/2(T) -> PS/2(T TID1)
  Feature extraction/1(R) -> PS/1(R TID1)
  Bus Selector/1 -> Feature extraction/1(Sig)  "<signal1>"
